simulink model "Test_Receive_CAN_V2"  (Simulink 7.0)
settings: Solver=FixedStepDiscrete  StartTime=0.0  StopTime=inf  FixedStep=0.025  RelTol=1e-3
settings Model: Creator=ilMaggia  LastModifiedBy=ilMaggia
settings DebuggingCC: SaveWithParameterizedLinksMsg=none  SignalResolutionControl=TryResolveAllWithWarning  MultiTaskDSMMsg=warning  MultiTaskCondExecSysMsg=none
settings RTWCC: SystemTargetFile=rtwin.tlc  TemplateMakefile=rtwin.tmf  Description=Real-Time Windows Target  ProcessScript=rtwin_make_rtw_hook  IncludeERTFirstTime=on
settings RTWinTargetCC: TargetFcnLib=ansi_tfl_tmw.mat  GenFloatMathFcnCalls=ANSI_C  ModelReferenceCompliant=off  CompOptLevelCompliant=off  PortableWordSizes=off  CCOptimize=on

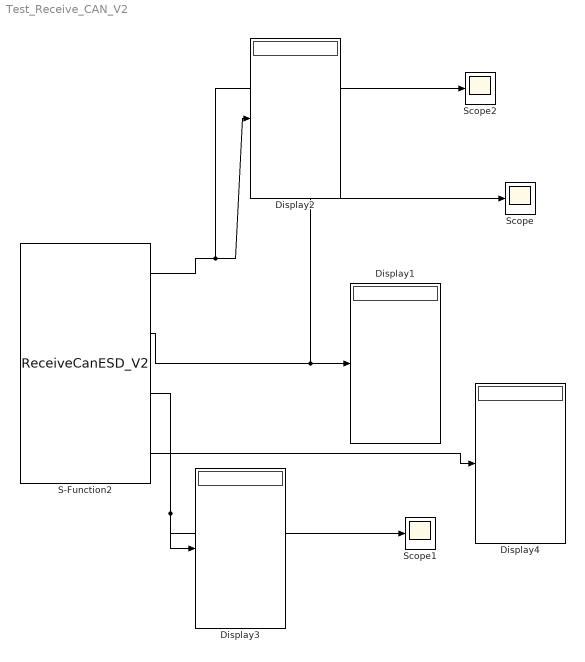
== system Test_Receive_CAN_V2 ==
  Display{1..4} (4 alike) : Display
  S-Function2 : S-Function  FunctionName=ReceiveCanESD_V2  Parameters=(baudrate),msgID  mask{msgID=[1365 1366 1367 43], baudrate=1000 Kbits/s}
      mask prompts: msgID "Message ID"
      mask StyleString: edit,popup(1000 Kbits/s|800  Kbits/s|666.6Kbits/s|500  Kbits/s)
      mask Display:
      | fprintf('RECEIVE CAN\n')
      | fprintf('\nID %d',msgID);
  Scope : Scope
      settings: YMin=0  YMax=3
  Scope1 : Scope
      settings: YMin=-100  YMax=1400
  Scope2 : Scope
      settings: YMin=0  YMax=275  SaveName=ScopeData2
  wires:
  S-Function2/1 -> Display2/1, Scope2/1
  S-Function2/2 -> Display1/1, Scope/1
  S-Function2/3 -> Display3/1, Scope1/1
  S-Function2/4 -> Display4/1
